simulink model "subscriber_udp_simulink"  (R2020a)
settings: Solver=VariableStepAuto  StartTime=0.0  StopTime=20  RelTol=1e-3
libraries: slrtlib x4, xpcutilitieslib x1, sldrtlib x1, xpcrtudplib x1
settings Model: EnablePacing=on  Creator=NGV-05  LastModifiedBy=AIMS_Zehui
settings DataIOCC: ReturnWorkspaceOutputs=off
settings DebuggingCC: ArithmeticOperatorsInVariantConditions=warning
settings SFSimCC: SimUseLocalCustomCode=off  CustomCodeUndefinedFunction=UseInterfaceOnly
settings RTWCC: RTWUseLocalCustomCode=off

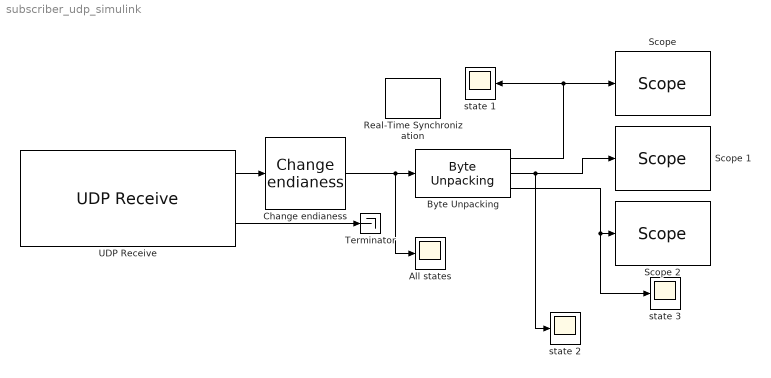
== system subscriber_udp_simulink ==
  All states : Scope
  "Byte Unpacking " : xpcutilitieslib/Byte Unpacking   MaskUnpackedDataTypes={'double','double','double'}  MaskUnpackedDataSizes={[1],[1],[1]}  MaskAlignment=8
      settings: SourceProductBaseCode=XP
  "Change endianess " : slrtlib/Shared Memory/Change endianess   numInp=1  lengthIn=Byte
      settings: SourceProductBaseCode=XP
  Real-Time Synchronization : sldrtlib/Real-Time Synchronization  SampleTime=0.1  MaxMissedTicks=10  ShowMissedTicks=off  YieldWhenWaiting=off
  "Scope " : slrtlib/Displays and Logging/Scope   scopeno=1  scopetype=Target  autostart=on  viewmode=Graphical redraw  formatstr='%15.6f'  grid=on  ylimits=[0,0]  nosamples=250  noprepostsamples=0  interleave=1  triggermode=FreeRun  triggersignal=1  trigsignalfromport=off  triggerlevel=0.0  triggerslope=Either  triggerscope=1  triggersample=0  filename=data.dat  mode=Lazy  writesize=512  autorestart=off  dynamicfilemode=off  maxwritefilesize=512*1024^2
  Scope 1 : slrtlib/Displays and Logging/Scope   scopeno=2  scopetype=Target  autostart=on  viewmode=Graphical redraw  formatstr='%15.6f'  grid=on  ylimits=[0,0]  nosamples=250  noprepostsamples=0  interleave=1  triggermode=FreeRun  triggersignal=1  trigsignalfromport=off  triggerlevel=0.0  triggerslope=Either  triggerscope=1  triggersample=0  filename=data.dat  mode=Lazy  writesize=512  autorestart=off  dynamicfilemode=off  maxwritefilesize=512*1024^2
  Scope 2 : slrtlib/Displays and Logging/Scope   scopeno=3  scopetype=Target  autostart=on  viewmode=Graphical redraw  formatstr='%15.6f'  grid=on  ylimits=[0,0]  nosamples=250  noprepostsamples=0  interleave=1  triggermode=FreeRun  triggersignal=1  trigsignalfromport=off  triggerlevel=0.0  triggerslope=Either  triggerscope=1  triggersample=0  filename=data.dat  mode=Lazy  writesize=512  autorestart=off  dynamicfilemode=off  maxwritefilesize=512*1024^2
  Terminator : Terminator
  UDP Receive : xpcrtudplib/UDP Receive  ipAddressVal=Use host-target connection  localPort=15005  rcvWidth=24  rcvFmAny=on  fmAddress=169.254.223.118  rcvMulticast=off  multicastAddress=[]  maxUDPQueue=8  sampleTime=-1
  state 1 : Scope
  state 2 : Scope
  state 3 : Scope
  wires:
  UDP Receive/2 -> Terminator/1
  UDP Receive/1 -> "Change endianess "/1
  "Byte Unpacking "/1 -> "Scope "/1, state 1/1
  "Byte Unpacking "/2 -> state 2/1, Scope 1/1
  "Byte Unpacking "/3 -> state 3/1, Scope 2/1
  "Change endianess "/1 -> All states/1, "Byte Unpacking "/1
